simulink model "ControlVehiculoElectrico"  (R2015a)
settings: Solver=ode23s  StartTime=0.0  StopTime=10.0  RelTol=1e-3
values from neighbouring files (symbols this model uses):
  J = Jv+Jw+J1    (= 0.629243511638)    [VehiculoElectrico.m]
  Kbm = 1/((pi/30)*Kb)    (= 0.19098593171)    [VehiculoElectrico.m]
  Kpwm = 5    [VehiculoElectrico.m]
  Ktm = (0.1130)*Kt    (= 0.1808)    [VehiculoElectrico.m]
  La = 0.1e-3    (= 0.0001)    [VehiculoElectrico.m]
  n = 3    [VehiculoElectrico.m]
  Ra = 0.013    [VehiculoElectrico.m]
  Ts = 6.6666e-5    (= 6.6666e-05)    [VehiculoElectrico.m]
libraries: cstblocks x2
settings Model: Creator=luis_  LastModifiedBy=luis_
settings SolverCC: ShapePreserveControl=EnableAll

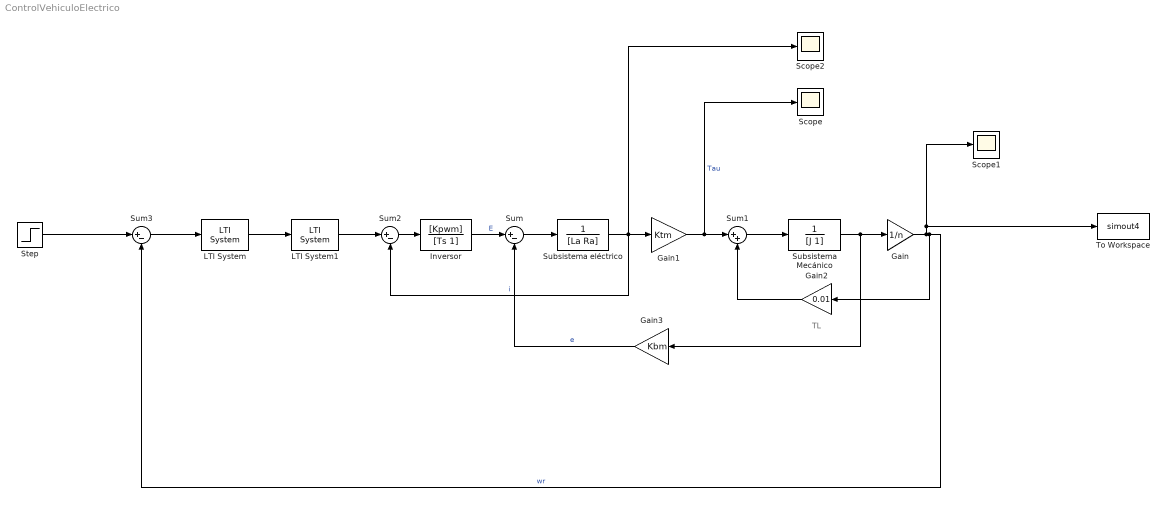
== system ControlVehiculoElectrico ==
  note: TL
  Gain : Gain  Gain=1/n
  Gain1 : Gain  Gain=Ktm
  Gain2 : Gain  Gain=0.01
  Gain3 : Gain  Gain=Kbm
  Inversor : TransferFcn  Numerator=[Kpwm]  Denominator=[Ts 1]
  LTI System : cstblocks/LTI System  sys=Gc1  IC=[]
  LTI System1 : cstblocks/LTI System  sys=PI  IC=[]
  Scope : Scope
  Scope1 : Scope
      settings: TimeRange=10
  Scope2 : Scope
      settings: YMin=1000  YMax=1000  SaveName=ScopeData2
  Step : Step  Time=0  After=455  SampleTime=0
  Subsistema Mecánico : TransferFcn  Denominator=[J 1]
  Subsistema eléctrico : TransferFcn  Denominator=[La Ra]
  Sum : Sum  Inputs=|+-
  Sum1 : Sum  Inputs=|++
  Sum2 : Sum  Inputs=|+-
  Sum3 : Sum  Inputs=|+-
  To Workspace : ToWorkspace  VariableName=simout4  SaveFormat=Timeseries  SampleTime=-1
  wires:
  Sum1/1 -> Subsistema Mecánico/1
  Subsistema Mecánico/1 -> Gain3/1, Gain/1
  Gain/1 -> Sum3/2, Gain2/1, To Workspace/1, Scope1/1  "wr"
  Inversor/1 -> Sum/1  "E"
  Sum/1 -> Subsistema eléctrico/1
  Subsistema eléctrico/1 -> Sum2/2, Scope2/1, Gain1/1  "i"
  Gain1/1 -> Scope/1, Sum1/1  "Tau"
  Gain3/1 -> Sum/2  "e"
  Gain2/1 -> Sum1/2
  Step/1 -> Sum3/1
  Sum3/1 -> LTI System/1
  Sum2/1 -> Inversor/1
  LTI System/1 -> LTI System1/1
  LTI System1/1 -> Sum2/1
